simulink model "Group44PACEMAKER"  (R2022b)
settings: Solver=FixedStepAuto  StartTime=0.0  StopTime=2  FixedStep=1e-2  RelTol=1e-3  EnableMultiTasking=on
undefined symbols (not defined in the file): D0, D1, D10, D11, D12, D13, D2, D3, D4, D5, D6, D7, D8, D9, PTA0, PTA1, PTA2, PTB23, PTB9, PTC16, PTC17, PTC2, PTC3, PTC4, PTD0, PTD1, PTD2, PTD3
libraries: frdmk64flib x15, dsparch4 x1, dspstat3 x1
(part 1 of 2)
settings Model: ExtModeTrigDuration=5  Creator=Admin  LastModifiedBy=Admin
settings OptimizationCC: EnhancedBackFolding=on  PassReuseOutputArgsAs=Individual arguments  ZeroExternalMemoryAtStartup=off  ZeroInternalMemoryAtStartup=off  MaxStackSize=64  OptimizeBlockOrder=speed  DifferentSizesBufferReuse=on  OptimizationCustomize=off  EfficientTunableParamExpr=on
settings DebuggingCC: ParameterTunabilityLossMsg=error
settings HardwareCC: ProdBitPerPointer=32  ProdBitPerSizeT=32  ProdBitPerPtrDiffT=32  ProdLargestAtomicInteger=Long  ProdLargestAtomicFloat=Double  ProdWordSize=32  ProdHWDeviceType=ARM Compatible->ARM Cortex
settings SFSimCC: MATLABDynamicMemAlloc=off
settings RTWCC: Description=Embedded Coder  SystemTargetFile=ert.tlc  HardwareBoard=NXP FRDM-K64F  TLCOptions="-aInlineSetEventsForThisBaseRateFcn=TLC_FALSE -aSuppressMultiTaskScheduler=TLC_FALSE  -aRateBasedStepFcn=0"  TemplateMakefile=ert_default_tmf  Toolchain=GNU Tools for ARM Embedded Processors
settings CodeAppCC: ForceParamTrailComments=on  IgnoreCustomStorageClasses=off  OperatorAnnotations=on  SimulinkDataObjDesc=on  SFDataObjDesc=on  InsertBlockDesc=on
settings ERTTargetCC: ExtModeTransport=4  ExtModeMexFile=sendToCommService

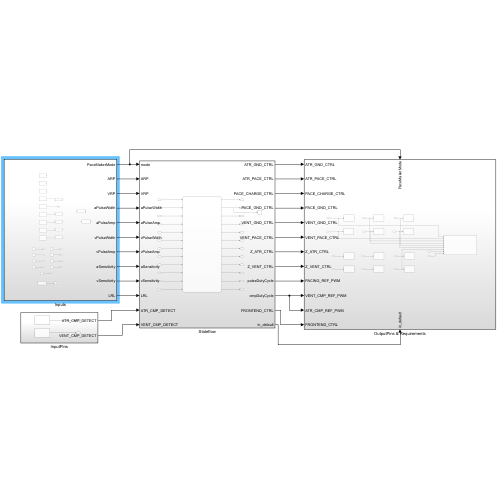
[thumbnail: Simulink's stored preview of the top-level diagram]
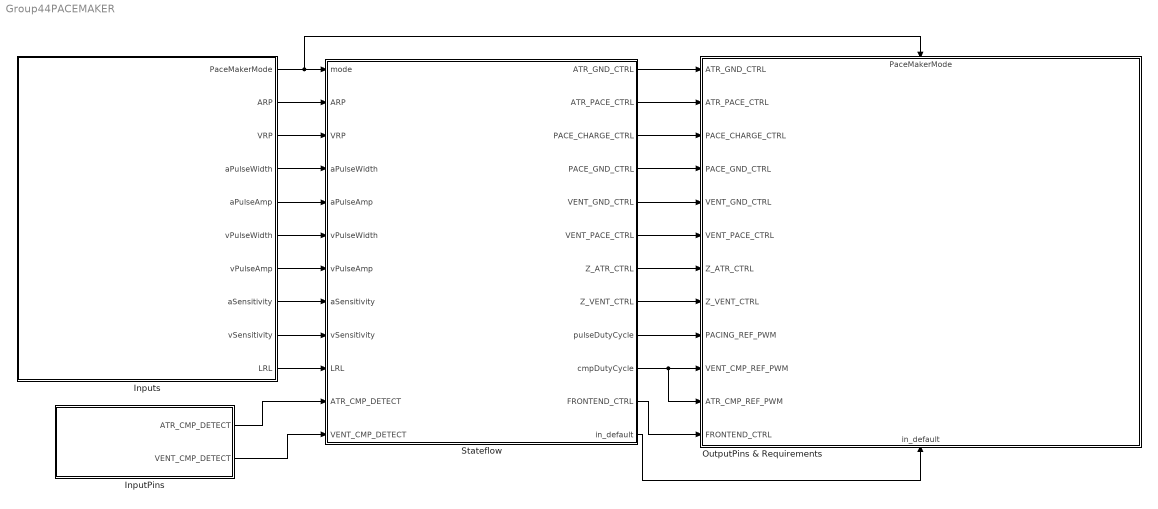
== system Group44PACEMAKER ==
  InputPins : Subsystem
  Inputs : Subsystem
  OutputPins & Requirements : Subsystem
      settings: PortSchema="{\"entries\":[{\"content\":{\"sides\":[{\"content\":{\"connectorIds\":[\"In1\",\"In2\",\"In3\",\"In4\",\"In5\",\"In6\",\"In7\",\"In8\",\"In9\",\"In10\",\"In11\",\"In12\"]},\"type\":\"ConnectorPlacement.EquallySpacedRectSide\",\"uuid\":\"f209b0ac-f79a-4701-a17d-e6e4657793a5\"},{\"content\":{\"connectorIds\":[],\"side\":\"RIGHT\"},\"type\":\"ConnectorPlacement.EquallySpacedRectSide\",\"uuid\":\"7d13a426-91e0-4712-bb01-5d8563f6962a\"},{\"content\":{\"connectorIds\":[\"In13\"],\"side\":\"TOP\"},\"type\":\"ConnectorPlacement.EquallySpacedRectSide\",\"uuid\":\"d5c2df9e-5684-45ec-bc45-fd2dab74cc87\"},{\"content\":{\"connectorIds\":[\"In14\"],\"side\":\"BOTTOM\"},\"type\":\"ConnectorPlacement.EquallySpacedRectSide\",\"uuid\":\"bae969d9-528a-49b4-ab28-7d9f0a0e5f3c\"}]},\"type\":\"ConnectorPlacement.EquallySpacedConnector\",\"uuid\":\"bb7a9bd2-ec42-4c9d-ad79-06266cd920c3\"}],\"packageUris\":[\"http://schema.mathworks.com/mf0/Connector/R2020b\"],\"version\":\"1.0\"}"
  Stateflow : Subsystem
  wires:
  Stateflow/12(in_default) -> OutputPins & Requirements/14(in_default)
  Stateflow/4(PACE_GND_CTRL) -> OutputPins & Requirements/4(PACE_GND_CTRL)
  Stateflow/10(cmpDutyCycle) -> OutputPins & Requirements/11(ATR_CMP_REF_PWM), OutputPins & Requirements/10(VENT_CMP_REF_PWM)
  Stateflow/5(VENT_GND_CTRL) -> OutputPins & Requirements/5(VENT_GND_CTRL)
  Stateflow/3(PACE_CHARGE_CTRL) -> OutputPins & Requirements/3(PACE_CHARGE_CTRL)
  InputPins/1(ATR_CMP_DETECT) -> Stateflow/11(ATR_CMP_DETECT)
  Stateflow/6(VENT_PACE_CTRL) -> OutputPins & Requirements/6(VENT_PACE_CTRL)
  Stateflow/2(ATR_PACE_CTRL) -> OutputPins & Requirements/2(ATR_PACE_CTRL)
  Stateflow/8(Z_VENT_CTRL) -> OutputPins & Requirements/8(Z_VENT_CTRL)
  Inputs/8(aSensitivity) -> Stateflow/8(aSensitivity)
  Inputs/7(vPulseAmp) -> Stateflow/7(vPulseAmp)
  Stateflow/7(Z_ATR_CTRL) -> OutputPins & Requirements/7(Z_ATR_CTRL)
  InputPins/2(VENT_CMP_DETECT) -> Stateflow/12(VENT_CMP_DETECT)
  Inputs/10(LRL) -> Stateflow/10(LRL)
  Stateflow/9(pulseDutyCycle) -> OutputPins & Requirements/9(PACING_REF_PWM)
  Inputs/4(aPulseWidth) -> Stateflow/4(aPulseWidth)
  Inputs/9(vSensitivity) -> Stateflow/9(vSensitivity)
  Inputs/2(ARP) -> Stateflow/2(ARP)
  Inputs/1(PaceMakerMode) -> OutputPins & Requirements/13(PaceMakerMode), Stateflow/1(mode)
  Stateflow/11(FRONTEND_CTRL) -> OutputPins & Requirements/12(FRONTEND_CTRL)
  Inputs/3(VRP) -> Stateflow/3(VRP)
  Inputs/6(vPulseWidth) -> Stateflow/6(vPulseWidth)
  Stateflow/1(ATR_GND_CTRL) -> OutputPins & Requirements/1(ATR_GND_CTRL)
  Inputs/5(aPulseAmp) -> Stateflow/5(aPulseAmp)

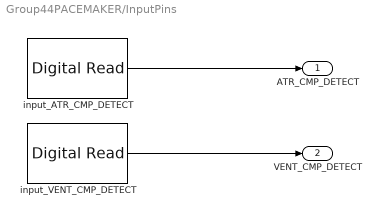
== system Group44PACEMAKER/InputPins ==
  input_ATR_CMP_DETECT : frdmk64flib/Digital Read  Whichpin=PTC16 (D0)  SampleTime=-1
  input_VENT_CMP_DETECT : frdmk64flib/Digital Read  Whichpin=PTC17 (D1)  SampleTime=-1
  ATR_CMP_DETECT : Outport  OutDataTypeStr=boolean
  VENT_CMP_DETECT : Outport  Port=2  OutDataTypeStr=boolean
  wires:
  input_ATR_CMP_DETECT/1 -> ATR_CMP_DETECT/1
  input_VENT_CMP_DETECT/1 -> VENT_CMP_DETECT/1

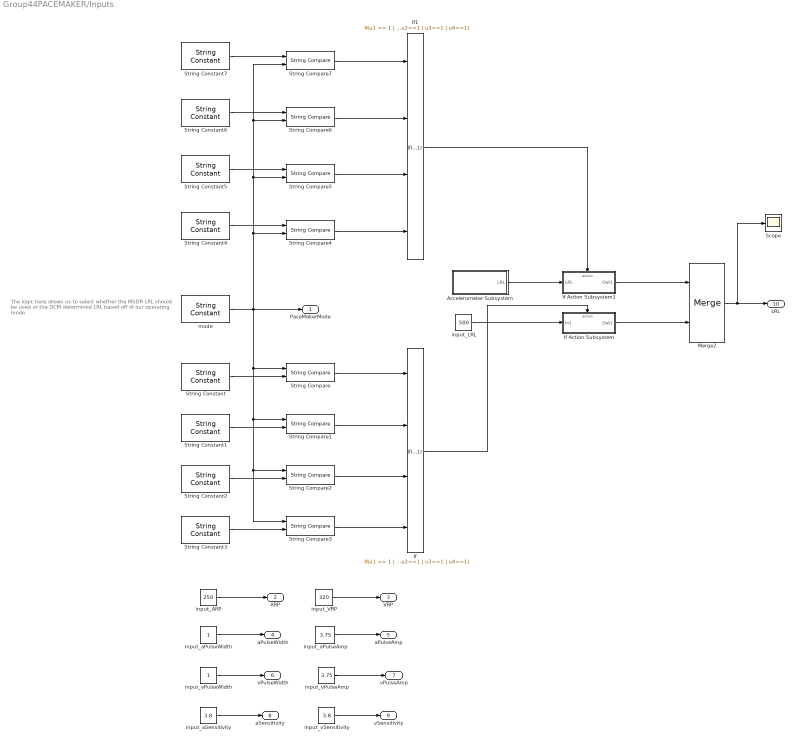
== system Group44PACEMAKER/Inputs ==
  note: The logic here allows us to select whether the MSDR LRL should be used or the DCM determined LRL based off of our operating mode
  Accelerometer Subsystem : Subsystem
  If : If  NumInputs=4  IfExpression=u1 == 1 | u2==1 | u3==1 | u4==1  ShowElse=off
  If Action Subsystem : Subsystem  TreatAsAtomicUnit=on
  If Action Subsystem1 : Subsystem  TreatAsAtomicUnit=on
  If1 : If  NumInputs=4  IfExpression=u1 == 1 | u2==1 | u3==1 | u4==1  ShowElse=off
  Merge2 : Merge
  Scope : Scope
  String Compare{,1..7} (8 alike) : StringCompare
  String Constant : StringConstant  String="\"AOO\""
  String Constant1 : StringConstant  String="\"AAI\""
  String Constant2 : StringConstant  String="\"VOO\""
  String Constant3 : StringConstant  String="\"VVI\""
  String Constant4 : StringConstant  String="\"AOOR\""
  String Constant5 : StringConstant  String="\"AAIR\""
  String Constant6 : StringConstant  String="\"VOOR\""
  String Constant7 : StringConstant  String="\"VVIR\""
  input_ARP : Constant  Value=250  OutDataTypeStr=double
  input_LRL : Constant  Value=500  OutDataTypeStr=double
  input_VRP : Constant  Value=320  OutDataTypeStr=double
  input_aPulseAmp : Constant  Value=3.75  OutDataTypeStr=double
  input_aPulseWidth : Constant  OutDataTypeStr=double
  input_aSensitivity : Constant  Value=3.8  OutDataTypeStr=double
  input_vPulseAmp : Constant  Value=3.75  OutDataTypeStr=double
  input_vPulseWidth : Constant  OutDataTypeStr=double
  input_vSensitivity : Constant  Value=3.8  OutDataTypeStr=double
  mode : StringConstant  String="\"AOOR\""
  PaceMakerMode : Outport  OutDataTypeStr=string
  ARP : Outport  Port=2  OutDataTypeStr=double  Unit=msec
  VRP : Outport  Port=3  OutDataTypeStr=double  Unit=msec
  aPulseWidth : Outport  Port=4  OutDataTypeStr=double  Unit=msec
  aPulseAmp : Outport  Port=5  OutDataTypeStr=double  Unit=V
  vPulseWidth : Outport  Port=6  OutDataTypeStr=double  Unit=msec
  vPulseAmp : Outport  Port=7  OutDataTypeStr=double  Unit=V
  aSensitivity : Outport  Port=8  OutDataTypeStr=double  Unit=V
  vSensitivity : Outport  Port=9  OutDataTypeStr=double  Unit=V
  LRL : Outport  Port=10  OutDataTypeStr=double  Unit=msec
  wires:
  mode/1 -> String Compare7/2, String Compare6/2, String Compare5/2, String Compare4/2, String Compare1/1, String Compare2/1, String Compare3/1, String Compare/1, PaceMakerMode/1
  input_aPulseAmp/1 -> aPulseAmp/1
  input_ARP/1 -> ARP/1
  input_VRP/1 -> VRP/1
  input_aPulseWidth/1 -> aPulseWidth/1
  input_vPulseWidth/1 -> vPulseWidth/1
  input_vPulseAmp/1 -> vPulseAmp/1
  input_vSensitivity/1 -> vSensitivity/1
  input_aSensitivity/1 -> aSensitivity/1
  String Constant/1 -> String Compare/2
  String Constant1/1 -> String Compare1/2
  String Constant2/1 -> String Compare2/2
  String Constant3/1 -> String Compare3/2
  String Constant4/1 -> String Compare4/1
  String Constant5/1 -> String Compare5/1
  String Constant6/1 -> String Compare6/1
  String Constant7/1 -> String Compare7/1
  If/1 -> If Action Subsystem/Action
  input_LRL/1 -> If Action Subsystem/1(In1)
  Merge2/1 -> Scope/1, LRL/1
  If Action Subsystem/1(Out1) -> Merge2/2
  If Action Subsystem1/1(Out1) -> Merge2/1
  String Compare3/1 -> If/4
  String Compare2/1 -> If/3
  String Compare1/1 -> If/2
  String Compare/1 -> If/1
  Accelerometer Subsystem/1(LRL) -> If Action Subsystem1/1(LRL)
  String Compare7/1 -> If1/1
  String Compare6/1 -> If1/2
  String Compare5/1 -> If1/3
  String Compare4/1 -> If1/4
  If1/1 -> If Action Subsystem1/Action

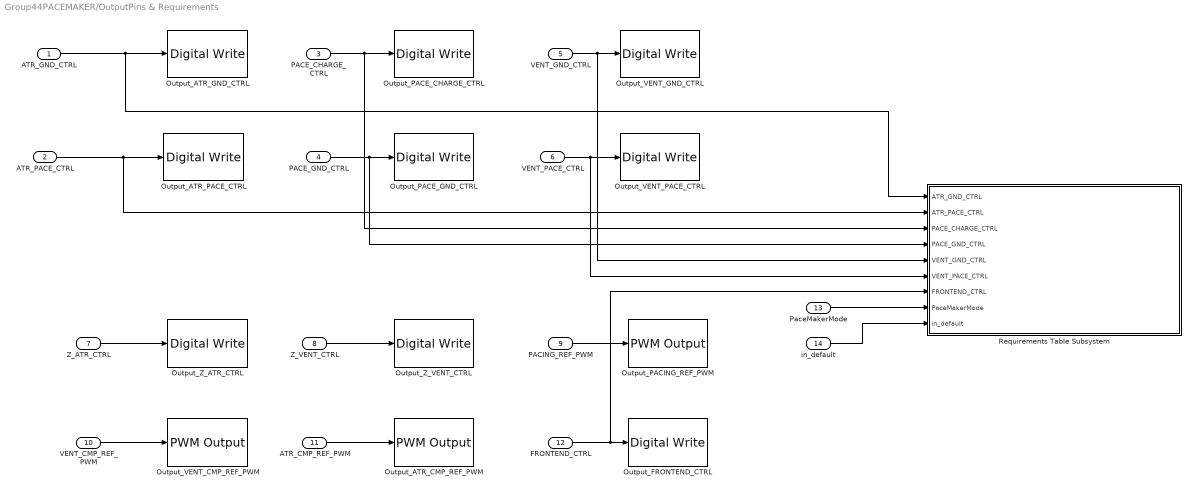
== system Group44PACEMAKER/OutputPins & Requirements ==
  ATR_GND_CTRL : Inport  OutDataTypeStr=boolean
  ATR_PACE_CTRL : Inport  Port=2  OutDataTypeStr=boolean
  PACE_CHARGE_CTRL : Inport  Port=3  OutDataTypeStr=boolean
  PACE_GND_CTRL : Inport  Port=4  OutDataTypeStr=boolean
  VENT_GND_CTRL : Inport  Port=5  OutDataTypeStr=boolean
  VENT_PACE_CTRL : Inport  Port=6  OutDataTypeStr=boolean
  Z_ATR_CTRL : Inport  Port=7  OutDataTypeStr=boolean
  Z_VENT_CTRL : Inport  Port=8  OutDataTypeStr=boolean
  PACING_REF_PWM : Inport  Port=9  OutDataTypeStr=double
  VENT_CMP_REF_PWM : Inport  Port=10  OutDataTypeStr=double
  ATR_CMP_REF_PWM : Inport  Port=11  OutDataTypeStr=double
  FRONTEND_CTRL : Inport  Port=12  OutDataTypeStr=boolean
  PaceMakerMode : Inport  Port=13  OutDataTypeStr=string
  in_default : Inport  Port=14  OutDataTypeStr=boolean
  Output_ATR_CMP_REF_PWM : frdmk64flib/PWM Output  Whichpin=PTC2 (D6)  InitialFrequency=2000  InitialDutyCycle=0
  Output_ATR_GND_CTRL : frdmk64flib/Digital Write  Whichpin=PTD2 (D11)
  Output_ATR_PACE_CTRL : frdmk64flib/Digital Write  Whichpin=PTA0 (D8)
  Output_FRONTEND_CTRL : frdmk64flib/Digital Write  Whichpin=PTD1 (D13)
  Output_PACE_CHARGE_CTRL : frdmk64flib/Digital Write  Whichpin=PTB9 (D2)
  Output_PACE_GND_CTRL : frdmk64flib/Digital Write  Whichpin=PTD0 (D10)
  Output_PACING_REF_PWM : frdmk64flib/PWM Output  Whichpin=PTA2 (D5)  InitialFrequency=2000  InitialDutyCycle=0
  Output_VENT_CMP_REF_PWM : frdmk64flib/PWM Output  Whichpin=PTA1 (D3)  InitialFrequency=2000  InitialDutyCycle=0
  Output_VENT_GND_CTRL : frdmk64flib/Digital Write  Whichpin=PTD3 (D12)
  Output_VENT_PACE_CTRL : frdmk64flib/Digital Write  Whichpin=PTC4 (D9)
  Output_Z_ATR_CTRL : frdmk64flib/Digital Write  Whichpin=PTB23 (D4)
  Output_Z_VENT_CTRL : frdmk64flib/Digital Write  Whichpin=PTC3 (D7)
  Requirements Table Subsystem : Subsystem
  wires:
  ATR_GND_CTRL/1 -> Requirements Table Subsystem/1(ATR_GND_CTRL), Output_ATR_GND_CTRL/1
  PACE_CHARGE_CTRL/1 -> Requirements Table Subsystem/3(PACE_CHARGE_CTRL), Output_PACE_CHARGE_CTRL/1
  VENT_GND_CTRL/1 -> Requirements Table Subsystem/5(VENT_GND_CTRL), Output_VENT_GND_CTRL/1
  VENT_PACE_CTRL/1 -> Requirements Table Subsystem/6(VENT_PACE_CTRL), Output_VENT_PACE_CTRL/1
  PACE_GND_CTRL/1 -> Requirements Table Subsystem/4(PACE_GND_CTRL), Output_PACE_GND_CTRL/1
  ATR_PACE_CTRL/1 -> Requirements Table Subsystem/2(ATR_PACE_CTRL), Output_ATR_PACE_CTRL/1
  Z_ATR_CTRL/1 -> Output_Z_ATR_CTRL/1
  Z_VENT_CTRL/1 -> Output_Z_VENT_CTRL/1
  PACING_REF_PWM/1 -> Output_PACING_REF_PWM/1
  ATR_CMP_REF_PWM/1 -> Output_ATR_CMP_REF_PWM/1
  VENT_CMP_REF_PWM/1 -> Output_VENT_CMP_REF_PWM/1
  FRONTEND_CTRL/1 -> Output_FRONTEND_CTRL/1, Requirements Table Subsystem/7(FRONTEND_CTRL)
  PaceMakerMode/1 -> Requirements Table Subsystem/8(PaceMakerMode)
  in_default/1 -> Requirements Table Subsystem/9(in_default)

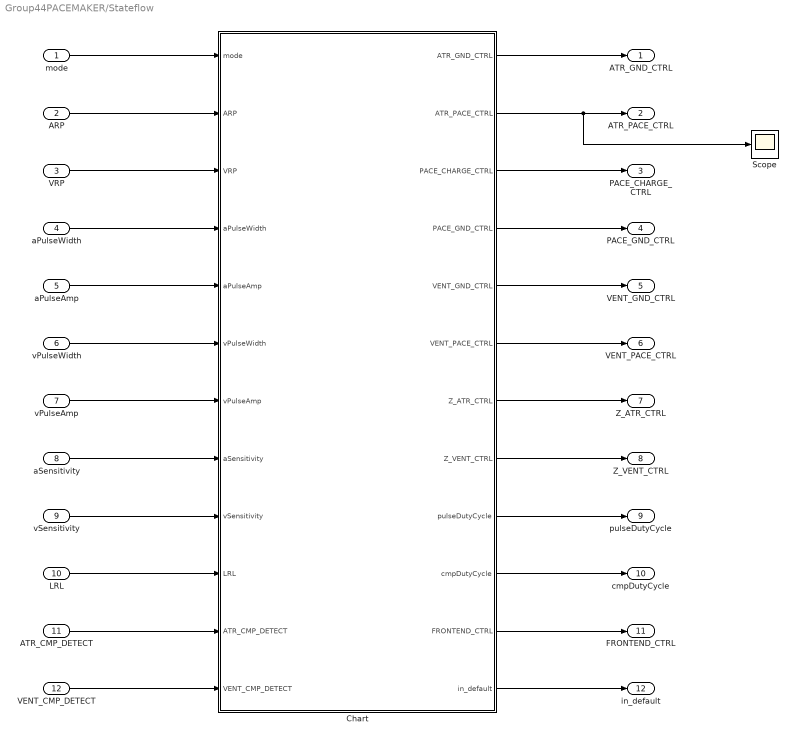
== system Group44PACEMAKER/Stateflow ==
  mode : Inport  OutDataTypeStr=string
  ARP : Inport  Port=2  OutDataTypeStr=double  Unit=msec
  VRP : Inport  Port=3  OutDataTypeStr=double  Unit=msec
  aPulseWidth : Inport  Port=4  OutDataTypeStr=double  Unit=msec
  aPulseAmp : Inport  Port=5  OutDataTypeStr=double  Unit=V
  vPulseWidth : Inport  Port=6  OutDataTypeStr=double  Unit=msec
  vPulseAmp : Inport  Port=7  OutDataTypeStr=double  Unit=V
  aSensitivity : Inport  Port=8  OutDataTypeStr=double  Unit=V
  vSensitivity : Inport  Port=9  OutDataTypeStr=double  Unit=V
  LRL : Inport  Port=10  OutDataTypeStr=double  Unit=msec
  ATR_CMP_DETECT : Inport  Port=11  OutDataTypeStr=boolean
  VENT_CMP_DETECT : Inport  Port=12  OutDataTypeStr=boolean
  Chart : Stateflow chart  TreatAsAtomicUnit=on
      settings: PortSchema="{\"entries\":[{\"content\":{\"sides\":[{\"content\":{\"connectorIds\":[\"In1\",\"In2\",\"In3\",\"In4\",\"In5\",\"In6\",\"In7\",\"In8\",\"In9\",\"In10\",\"In11\",\"In12\"]},\"type\":\"ConnectorPlacement.EquallySpacedRectSide\",\"uuid\":\"859ad6b1-f88a-4c7a-b788-dab0771a046c\"},{\"content\":{\"connectorIds\":[\"Out1\",\"Out2\",\"Out4\",\"Out5\",\"Out6\",\"Out7\",\"Out8\",\"Out9\",\"Out12\",\"Out10\",\"Out3\",\"Out11\"],\"side\":\"RIGHT\"},\"type\":\"ConnectorPlacement.EquallySpacedRectSide\",\"uuid\":\"6cbb226c-0635-41e8-91ac-a9d01d96dd8d\"},{\"content\":{\"connectorIds\":[],\"side\":\"TOP\"},\"type\":\"ConnectorPlacement.EquallySpacedRectSide\",\"uuid\":\"47ebdae6-f6ae-4f62-b33d-fff46319b1f0\"}]},\"type\":\"ConnectorPlacement.EquallySpacedConnector\",\"uuid\":\"c5e573a1-920d-4865-9b5e-320d436c45e0\"}],\"packageUris\":[\"http://schema.mathworks.com/mf0/Connector/R2020b\"],\"version\":\"1.0\"}"
  Scope : Scope
  ATR_GND_CTRL : Outport  OutDataTypeStr=boolean
  ATR_PACE_CTRL : Outport  Port=2  OutDataTypeStr=boolean
  PACE_CHARGE_CTRL : Outport  Port=3  OutDataTypeStr=boolean
  PACE_GND_CTRL : Outport  Port=4  OutDataTypeStr=boolean
  VENT_GND_CTRL : Outport  Port=5  OutDataTypeStr=boolean
  VENT_PACE_CTRL : Outport  Port=6  OutDataTypeStr=boolean
  Z_ATR_CTRL : Outport  Port=7  OutDataTypeStr=boolean
  Z_VENT_CTRL : Outport  Port=8  OutDataTypeStr=boolean
  pulseDutyCycle : Outport  Port=9  OutDataTypeStr=double
  cmpDutyCycle : Outport  Port=10  OutDataTypeStr=double
  FRONTEND_CTRL : Outport  Port=11  OutDataTypeStr=boolean
  in_default : Outport  Port=12  OutDataTypeStr=boolean
  wires:
  mode/1 -> Chart/1(mode)
  ARP/1 -> Chart/2(ARP)
  VRP/1 -> Chart/3(VRP)
  aPulseWidth/1 -> Chart/4(aPulseWidth)
  aPulseAmp/1 -> Chart/5(aPulseAmp)
  vPulseWidth/1 -> Chart/6(vPulseWidth)
  vPulseAmp/1 -> Chart/7(vPulseAmp)
  aSensitivity/1 -> Chart/8(aSensitivity)
  vSensitivity/1 -> Chart/9(vSensitivity)
  LRL/1 -> Chart/10(LRL)
  ATR_CMP_DETECT/1 -> Chart/11(ATR_CMP_DETECT)
  VENT_CMP_DETECT/1 -> Chart/12(VENT_CMP_DETECT)
  Chart/1(ATR_GND_CTRL) -> ATR_GND_CTRL/1
  Chart/2(ATR_PACE_CTRL) -> Scope/1, ATR_PACE_CTRL/1
  Chart/4(PACE_CHARGE_CTRL) -> PACE_CHARGE_CTRL/1
  Chart/5(PACE_GND_CTRL) -> PACE_GND_CTRL/1
  Chart/6(VENT_GND_CTRL) -> VENT_GND_CTRL/1
  Chart/7(VENT_PACE_CTRL) -> VENT_PACE_CTRL/1
  Chart/8(Z_ATR_CTRL) -> Z_ATR_CTRL/1
  Chart/9(Z_VENT_CTRL) -> Z_VENT_CTRL/1
  Chart/10(cmpDutyCycle) -> cmpDutyCycle/1
  Chart/3(FRONTEND_CTRL) -> FRONTEND_CTRL/1
  Chart/11(in_default) -> in_default/1
  Chart/12(pulseDutyCycle) -> pulseDutyCycle/1

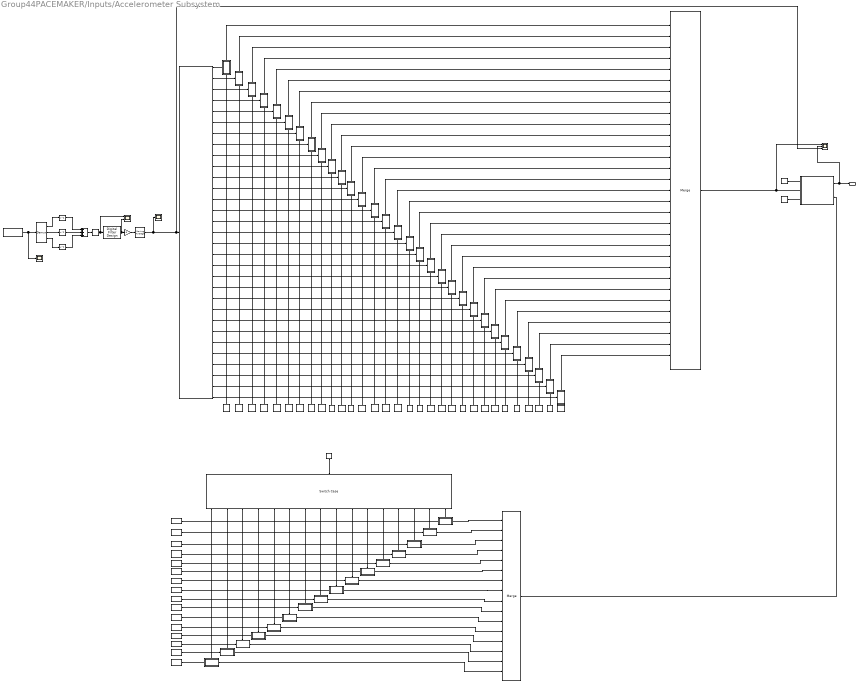
== system Group44PACEMAKER/Inputs/Accelerometer Subsystem ==
  note: The chart allows us to come up with a steady rate of change for the heart LRL such that the heart rate changes smoothly over the reaction time/recovery time
  note: This if else block allows us to select the appropriate LRL based on activity level
  note: The squared terms, adder, and square root term allow us to get the magnitude of the acceleration vector
  note: Moving average smooths out activity level and allows us to average out the activity for the past x seconds dependent of model fixed step time and the window used
  note: The gain function amplifies the signal so changes in activity can easily be observed using the scope
  note: The low pass filter gets rid of any intense spikes or dips that are not characterist of the activity
  note: The response factor can range from 1 to 16. 1 being the lowest response factor and 16 being the highest.
      | The response factor is used to determine a percentage of the of the reaction time that will be used to adjust the LRL. (Eg, a response factor of 1 will use 100% of the reaction time however a response factor of 16 will only use 70% of the reaction time)
  100 bpm : Constant  Value=600
  105 bpm : Constant  Value=571.43
  110 bpm : Constant  Value=545.45
  115 bpm : Constant  Value=521.74
  120 bpm : Constant  Value=500
  125 bpm : Constant  Value=480
  130 bpm : Constant  Value=461.54
  135 bpm : Constant  Value=444.44
  140 bpm : Constant  Value=428.57
  145 bpm : Constant  Value=413.79
  150 bpm : Constant  Value=400
  155 bpm : Constant  Value=387.10
  160 bpm : Constant  Value=375
  165 bpm : Constant  Value=363.63
  170 bpm1 : Constant  Value=352.94
  175 bpm : Constant  Value=342.86
  180 bpm : Constant  Value=333.33
  185 bpm : Constant  Value=324.32
  190 bpm : Constant  Value=315.79
  195 bpm : Constant  Value=307.69
  200 bpm : Constant  Value=300
  205 bpm : Constant  Value=292.68
  55 bpm : Constant  Value=1090.91
  60 bpm : Constant  Value=1000
  65 bpm : Constant  Value=923.08
  70 bpm : Constant  Value=857.14
  75 bpm : Constant  Value=800
  80 bpm : Constant  Value=750
  85 bpm : Constant  Value=705.88
  90 bpm : Constant  Value=666.67
  95 bpm : Constant  Value=631.58
  >7.9 : Subsystem  TreatAsAtomicUnit=on
  >8 : Subsystem  TreatAsAtomicUnit=on
  Accelerometer : Subsystem
  Add : Sum  Inputs=+++
  Change LRL Smoothly : Stateflow chart  TreatAsAtomicUnit=on
      settings: PortSchema="{\"entries\":[{\"content\":{\"sides\":[{\"content\":{\"connectorIds\":[\"In3\",\"In2\",\"In4\"]},\"type\":\"ConnectorPlacement.EquallySpacedRectSide\",\"uuid\":\"85af1beb-61ae-4766-b408-8225321ec4a4\"},{\"content\":{\"connectorIds\":[\"Out1\",\"In1\"],\"side\":\"RIGHT\"},\"type\":\"ConnectorPlacement.EquallySpacedRectSide\",\"uuid\":\"bdf3d147-5894-49ca-bdec-54ebdf64bfa8\"},{\"content\":{\"connectorIds\":[],\"side\":\"TOP\"},\"type\":\"ConnectorPlacement.EquallySpacedRectSide\",\"uuid\":\"42bc5e47-54de-4fed-b1f0-fe2ea6e0cd28\"},{\"content\":{\"connectorIds\":[],\"side\":\"BOTTOM\"},\"type\":\"ConnectorPlacement.EquallySpacedRectSide\",\"uuid\":\"092d377f-872f-4731-90ca-5dcd29f87b08\"}]},\"type\":\"ConnectorPlacement.EquallySpacedConnector\",\"uuid\":\"a2c4c5d6-6aa5-4141-8747-f931ac594277\"}],\"packageUris\":[\"http://schema.mathworks.com/mf0/Connector/R2020b\"],\"version\":\"1.0\"}"
  Demux : Demux  Outputs=3
      settings: DisplayOption=none
  Gain : Gain  Gain=5
  If : If  IfExpression=u1 > 8  ElseIfExpressions=u1>7.9, u1>7.8, u1>7.7, u1>7.6, u1>7.5, u1>7.4, u1>7.3, u1>7.2, u1>7.1, u1 > 7, u1>6.9, u1>6.8, u1>6.7, u1>6.6, u1>6.5, u1>6.4, u1>6.3, u1>6.2, u1>6.1, u1 >6, u1>5.9, u1>5.8, u1>5.7, u1>5.6, u1>5.5, u1>5.4, u1>5.3, u1>5.2, u1>5.1
  If Action Subsystem : Subsystem  TreatAsAtomicUnit=on
  If Action Subsystem1 : Subsystem  TreatAsAtomicUnit=on
  If Action Subsystem10 : Subsystem  TreatAsAtomicUnit=on
  If Action Subsystem11 : Subsystem  TreatAsAtomicUnit=on
  If Action Subsystem12 : Subsystem  TreatAsAtomicUnit=on
  If Action Subsystem13 : Subsystem  TreatAsAtomicUnit=on
  If Action Subsystem14 : Subsystem  TreatAsAtomicUnit=on
  If Action Subsystem15 : Subsystem  TreatAsAtomicUnit=on
  If Action Subsystem16 : Subsystem  TreatAsAtomicUnit=on
  If Action Subsystem17 : Subsystem  TreatAsAtomicUnit=on
  If Action Subsystem18 : Subsystem  TreatAsAtomicUnit=on
  If Action Subsystem19 : Subsystem  TreatAsAtomicUnit=on
  If Action Subsystem2 : Subsystem  TreatAsAtomicUnit=on
  If Action Subsystem20 : Subsystem  TreatAsAtomicUnit=on
  If Action Subsystem21 : Subsystem  TreatAsAtomicUnit=on
  If Action Subsystem22 : Subsystem  TreatAsAtomicUnit=on
  If Action Subsystem23 : Subsystem  TreatAsAtomicUnit=on
  If Action Subsystem24 : Subsystem  TreatAsAtomicUnit=on
  If Action Subsystem25 : Subsystem  TreatAsAtomicUnit=on
  If Action Subsystem26 : Subsystem  TreatAsAtomicUnit=on
  If Action Subsystem3 : Subsystem  TreatAsAtomicUnit=on
  If Action Subsystem4 : Subsystem  TreatAsAtomicUnit=on
  If Action Subsystem5 : Subsystem  TreatAsAtomicUnit=on
  If Action Subsystem6 : Subsystem  TreatAsAtomicUnit=on
  If Action Subsystem7 : Subsystem  TreatAsAtomicUnit=on
  If Action Subsystem8 : Subsystem  TreatAsAtomicUnit=on
  If Action Subsystem9 : Subsystem  TreatAsAtomicUnit=on
  LowPassFilter : dsparch4/Digital Filter Design  mwdsp_browser_bugfix_var=off
  Merge : Merge  Inputs=31
  Merge1 : Merge  Inputs=16
  Moderate activity LRL if subsystem : Subsystem  TreatAsAtomicUnit=on
  Moving Average1 : dspstat3/Moving Average  Method=Sliding window  ForgettingFactorPort=off  SpecifyWindowLength=on  WindowLength=500  OverlapLength=499  AllowArbitraryInputLength=off  ForgettingFactor=0.9  SimulateUsing=Code generation
  RF == 1 : Subsystem  TreatAsAtomicUnit=on
  RF == 10 : Subsystem  TreatAsAtomicUnit=on
  RF == 11 : Subsystem  TreatAsAtomicUnit=on
  RF == 12 : Subsystem  TreatAsAtomicUnit=on
  RF == 13 : Subsystem  TreatAsAtomicUnit=on
  RF == 14 : Subsystem  TreatAsAtomicUnit=on
  RF == 15 : Subsystem  TreatAsAtomicUnit=on
  RF == 16 : Subsystem  TreatAsAtomicUnit=on
  RF == 2 : Subsystem  TreatAsAtomicUnit=on
  RF == 3 : Subsystem  TreatAsAtomicUnit=on
  RF == 4 : Subsystem  TreatAsAtomicUnit=on
  RF == 5 : Subsystem  TreatAsAtomicUnit=on
  RF == 6 : Subsystem  TreatAsAtomicUnit=on
  RF == 7 : Subsystem  TreatAsAtomicUnit=on
  RF == 8 : Subsystem  TreatAsAtomicUnit=on
  RF == 9 : Subsystem  TreatAsAtomicUnit=on
  RF_1 : Constant  Value=100
  RF_10 : Constant  Value=82
  RF_11 : Constant  Value=80
  RF_12 : Constant  Value=78
  RF_13 : Constant  Value=76
  RF_14 : Constant  Value=74
  RF_15 : Constant  Value=72
  RF_16 : Constant  Value=70
  RF_2 : Constant  Value=98  OutDataTypeStr=double
  RF_3 : Constant  Value=96
  RF_4 : Constant  Value=94
  RF_5 : Constant  Value=92
  RF_6 : Constant  Value=90
  RF_7 : Constant  Value=88
  RF_8 : Constant  Value=86
  RF_9 : Constant  Value=84
  Response Factor Switch Case : SwitchCase  CaseConditions={1,2,3,4,5,6,7,8,9,10,11,12,13,14,15,16}  ShowDefaultCase=off
  Response_factor : Constant
  Scope : Scope  NumInputPorts=3
  Scope1 : Scope
  Scope2 : Scope  NumInputPorts=2
  Scope3 : Scope
  Square : Math  Operator=square
  Square Root : Sqrt
  Square1 : Math  Operator=square
  Square2 : Math  Operator=square
  Vigorous activity LRL if subsystem : Subsystem  TreatAsAtomicUnit=on
  reaction_time(sec) : Constant  Value=5
  recovery_time(min) : Constant  Value=.1
  LRL : Outport
  wires:
  Add/1 -> Square Root/1
  Gain/1 -> Moving Average1/1
  Square1/1 -> Add/2
  LowPassFilter/1 -> Scope2/2, Gain/1
  Square/1 -> Add/1
  Demux/2 -> Square1/1
  Accelerometer/1(Acceleration) -> Scope1/1, Demux/1
  Demux/3 -> Square2/1
  Demux/1 -> Square/1
  Square2/1 -> Add/3
  Square Root/1 -> Scope2/1, LowPassFilter/1
  Moving Average1/1 -> Scope3/1, Scope/3, If/1
  Merge/1 -> Scope/1, Change LRL Smoothly/2(inputLRL)
  Change LRL Smoothly/1(outputLRL) -> LRL/1, Scope/2
  reaction_time(sec)/1 -> Change LRL Smoothly/3(reaction_time)
  recovery_time(min)/1 -> Change LRL Smoothly/4(recovery_time)
  Response_factor/1 -> Response Factor Switch Case/1
  Response Factor Switch Case/2 -> RF == 2/Action
  Response Factor Switch Case/1 -> RF == 1/Action
  Response Factor Switch Case/3 -> RF == 3/Action
  Response Factor Switch Case/4 -> RF == 4/Action
  Response Factor Switch Case/5 -> RF == 5/Action
  Response Factor Switch Case/6 -> RF == 6/Action
  Response Factor Switch Case/7 -> RF == 7/Action
  Response Factor Switch Case/8 -> RF == 8/Action
  Response Factor Switch Case/9 -> RF == 9/Action
  Response Factor Switch Case/10 -> RF == 10/Action
  Response Factor Switch Case/11 -> RF == 11/Action
  Response Factor Switch Case/12 -> RF == 12/Action
  Response Factor Switch Case/13 -> RF == 13/Action
  Response Factor Switch Case/15 -> RF == 15/Action
  Response Factor Switch Case/14 -> RF == 14/Action
  Response Factor Switch Case/16 -> RF == 16/Action
  RF_1/1 -> RF == 1/1(In1)
  RF_3/1 -> RF == 3/1(In1)
  RF_2/1 -> RF == 2/1(In1)
  RF_4/1 -> RF == 4/1(In1)
  RF_5/1 -> RF == 5/1(In1)
  RF_6/1 -> RF == 6/1(In1)
  RF_7/1 -> RF == 7/1(In1)
  RF_8/1 -> RF == 8/1(In1)
  RF_9/1 -> RF == 9/1(In1)
  RF_10/1 -> RF == 10/1(In1)
  RF_11/1 -> RF == 11/1(In1)
  RF_12/1 -> RF == 12/1(In1)
  RF_13/1 -> RF == 13/1(In1)
  RF_14/1 -> RF == 14/1(In1)
  RF_15/1 -> RF == 15/1(In1)
  RF_16/1 -> RF == 16/1(In1)
  RF == 16/1(Out1) -> Merge1/1
  RF == 15/1(Out1) -> Merge1/2
  RF == 14/1(Out1) -> Merge1/3
  RF == 13/1(Out1) -> Merge1/4
  RF == 12/1(Out1) -> Merge1/5
  RF == 11/1(Out1) -> Merge1/6
  RF == 10/1(Out1) -> Merge1/7
  RF == 1/1(Out1) -> Merge1/16
  RF == 2/1(Out1) -> Merge1/15
  RF == 3/1(Out1) -> Merge1/14
  RF == 4/1(Out1) -> Merge1/13
  RF == 5/1(Out1) -> Merge1/12
  RF == 6/1(Out1) -> Merge1/11
  RF == 7/1(Out1) -> Merge1/10
  RF == 8/1(Out1) -> Merge1/9
  RF == 9/1(Out1) -> Merge1/8
  Merge1/1 -> Change LRL Smoothly/1(Response_factor)
  If/1 -> >8/Action
  If/2 -> >7.9/Action
  If/3 -> Moderate activity LRL if subsystem/Action
  If/4 -> Vigorous activity LRL if subsystem/Action
  If/5 -> If Action Subsystem/Action
  If/6 -> If Action Subsystem1/Action
  If/7 -> If Action Subsystem2/Action
  If/8 -> If Action Subsystem3/Action
  If/9 -> If Action Subsystem4/Action
  If/10 -> If Action Subsystem5/Action
  If/11 -> If Action Subsystem6/Action
  If/12 -> If Action Subsystem7/Action
  If/13 -> If Action Subsystem8/Action
  If/14 -> If Action Subsystem9/Action
  If/15 -> If Action Subsystem10/Action
  If/16 -> If Action Subsystem11/Action
  If/17 -> If Action Subsystem12/Action
  If/18 -> If Action Subsystem13/Action
  If/19 -> If Action Subsystem14/Action
  If/20 -> If Action Subsystem15/Action
  If/21 -> If Action Subsystem16/Action
  If/22 -> If Action Subsystem17/Action
  If/23 -> If Action Subsystem18/Action
  If/24 -> If Action Subsystem19/Action
  If/25 -> If Action Subsystem20/Action
  If/26 -> If Action Subsystem21/Action
  If/27 -> If Action Subsystem22/Action
  If/28 -> If Action Subsystem23/Action
  If/29 -> If Action Subsystem24/Action
  If/30 -> If Action Subsystem25/Action
  If/31 -> If Action Subsystem26/Action
  205 bpm/1 -> >8/1(In1)
  200 bpm/1 -> >7.9/1(In1)
  195 bpm/1 -> Moderate activity LRL if subsystem/1(In1)
  190 bpm/1 -> Vigorous activity LRL if subsystem/1(In1)
  185 bpm/1 -> If Action Subsystem/1(In1)
  180 bpm/1 -> If Action Subsystem1/1(In1)
  175 bpm/1 -> If Action Subsystem2/1(In1)
  170 bpm1/1 -> If Action Subsystem3/1(In1)
  165 bpm/1 -> If Action Subsystem4/1(In1)
  160 bpm/1 -> If Action Subsystem5/1(In1)
  155 bpm/1 -> If Action Subsystem6/1(In1)
  150 bpm/1 -> If Action Subsystem7/1(In1)
  145 bpm/1 -> If Action Subsystem8/1(In1)
  140 bpm/1 -> If Action Subsystem9/1(In1)
  135 bpm/1 -> If Action Subsystem10/1(In1)
  130 bpm/1 -> If Action Subsystem11/1(In1)
  125 bpm/1 -> If Action Subsystem12/1(In1)
  120 bpm/1 -> If Action Subsystem13/1(In1)
  115 bpm/1 -> If Action Subsystem14/1(In1)
  110 bpm/1 -> If Action Subsystem15/1(In1)
  105 bpm/1 -> If Action Subsystem16/1(In1)
  100 bpm/1 -> If Action Subsystem17/1(In1)
  95 bpm/1 -> If Action Subsystem18/1(In1)
  90 bpm/1 -> If Action Subsystem19/1(In1)
  85 bpm/1 -> If Action Subsystem20/1(In1)
  80 bpm/1 -> If Action Subsystem21/1(In1)
  75 bpm/1 -> If Action Subsystem22/1(In1)
  70 bpm/1 -> If Action Subsystem23/1(In1)
  65 bpm/1 -> If Action Subsystem24/1(In1)
  60 bpm/1 -> If Action Subsystem25/1(In1)
  55 bpm/1 -> If Action Subsystem26/1(In1)
  >8/1(Out1) -> Merge/1
  >7.9/1(Out1) -> Merge/2
  Moderate activity LRL if subsystem/1(Out1) -> Merge/3
  Vigorous activity LRL if subsystem/1(Out1) -> Merge/4
  If Action Subsystem/1(Out1) -> Merge/5
  If Action Subsystem1/1(Out1) -> Merge/6
  If Action Subsystem2/1(Out1) -> Merge/7
  If Action Subsystem3/1(Out1) -> Merge/8
  If Action Subsystem4/1(Out1) -> Merge/9
  If Action Subsystem5/1(Out1) -> Merge/10
  If Action Subsystem6/1(Out1) -> Merge/11
  If Action Subsystem7/1(Out1) -> Merge/12
  If Action Subsystem8/1(Out1) -> Merge/13
  If Action Subsystem9/1(Out1) -> Merge/14
  If Action Subsystem10/1(Out1) -> Merge/15
  If Action Subsystem11/1(Out1) -> Merge/16
  If Action Subsystem12/1(Out1) -> Merge/17
  If Action Subsystem13/1(Out1) -> Merge/18
  If Action Subsystem14/1(Out1) -> Merge/19
  If Action Subsystem15/1(Out1) -> Merge/20
  If Action Subsystem16/1(Out1) -> Merge/21
  If Action Subsystem17/1(Out1) -> Merge/22
  If Action Subsystem18/1(Out1) -> Merge/23
  If Action Subsystem19/1(Out1) -> Merge/24
  If Action Subsystem20/1(Out1) -> Merge/25
  If Action Subsystem21/1(Out1) -> Merge/26
  If Action Subsystem22/1(Out1) -> Merge/27
  If Action Subsystem23/1(Out1) -> Merge/28
  If Action Subsystem24/1(Out1) -> Merge/29
  If Action Subsystem25/1(Out1) -> Merge/30
  If Action Subsystem26/1(Out1) -> Merge/31

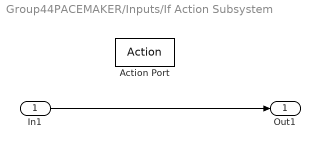
== system Group44PACEMAKER/Inputs/If Action Subsystem ==
  In1 : Inport
  Action Port : ActionPort  ActionPortLabel=if(u1 == 1 | u2==1 | u3==1 | u4==1)
  Out1 : Outport
  wires:
  In1/1 -> Out1/1

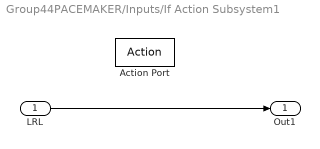
== system Group44PACEMAKER/Inputs/If Action Subsystem1 ==
  LRL : Inport
  Action Port : ActionPort  ActionPortLabel=if(u1 == 1 | u2==1 | u3==1 | u4==1)
  Out1 : Outport
  wires:
  LRL/1 -> Out1/1

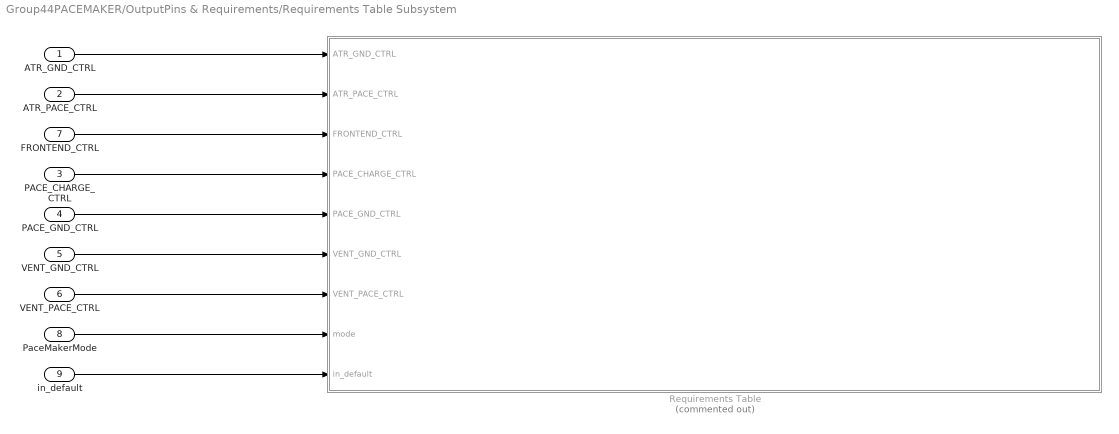
== system Group44PACEMAKER/OutputPins & Requirements/Requirements Table Subsystem ==
  ATR_GND_CTRL : Inport  OutDataTypeStr=boolean
  ATR_PACE_CTRL : Inport  Port=2  OutDataTypeStr=boolean
  PACE_CHARGE_CTRL : Inport  Port=3  OutDataTypeStr=boolean
  PACE_GND_CTRL : Inport  Port=4  OutDataTypeStr=boolean
  VENT_GND_CTRL : Inport  Port=5  OutDataTypeStr=boolean
  VENT_PACE_CTRL : Inport  Port=6  OutDataTypeStr=boolean
  FRONTEND_CTRL : Inport  Port=7  OutDataTypeStr=boolean
  PaceMakerMode : Inport  Port=8  OutDataTypeStr=string
  in_default : Inport  Port=9  OutDataTypeStr=boolean
  Requirements Table : Requirements Table  Commented=on  TreatAsAtomicUnit=on
  wires:
  ATR_GND_CTRL/1 -> Requirements Table/1(ATR_GND_CTRL)
  ATR_PACE_CTRL/1 -> Requirements Table/2(ATR_PACE_CTRL)
  PACE_CHARGE_CTRL/1 -> Requirements Table/4(PACE_CHARGE_CTRL)
  PACE_GND_CTRL/1 -> Requirements Table/5(PACE_GND_CTRL)
  VENT_GND_CTRL/1 -> Requirements Table/6(VENT_GND_CTRL)
  VENT_PACE_CTRL/1 -> Requirements Table/7(VENT_PACE_CTRL)
  FRONTEND_CTRL/1 -> Requirements Table/3(FRONTEND_CTRL)
  PaceMakerMode/1 -> Requirements Table/8(mode)
  in_default/1 -> Requirements Table/9(in_default)

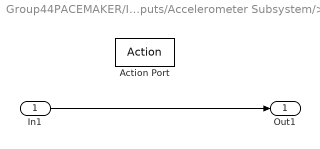
== system Group44PACEMAKER/Inputs/Accelerometer Subsystem/>7.9 ==
  In1 : Inport
  Action Port : ActionPort  ActionPortLabel=elseif(u1>7.9)
  Out1 : Outport
  wires:
  In1/1 -> Out1/1

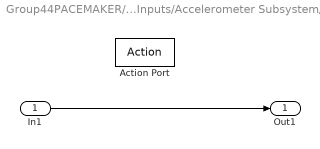
== system Group44PACEMAKER/Inputs/Accelerometer Subsystem/>8 ==
  In1 : Inport
  Action Port : ActionPort  ActionPortLabel=if(u1 > 8)
  Out1 : Outport
  wires:
  In1/1 -> Out1/1

== system Group44PACEMAKER/Inputs/Accelerometer Subsystem/Accelerometer ==
  FXOS8700 6-Axes Sensor : frdmk64flib/FXOS8700 6-Axes Sensor  Activesensor=Accelerometer only  ODR=800Hz  HybridODR=400Hz  Accelfullrange=-8g to +8g  SampleTime=-1
  Acceleration : Outport
  wires:
  FXOS8700 6-Axes Sensor/1 -> Acceleration/1

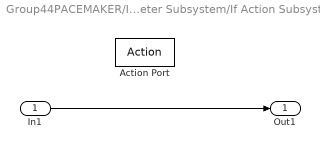
== system Group44PACEMAKER/Inputs/Accelerometer Subsystem/If Action Subsystem ==
  In1 : Inport
  Action Port : ActionPort  ActionPortLabel=elseif( u1>7.6)
  Out1 : Outport
  wires:
  In1/1 -> Out1/1

== system Group44PACEMAKER/Inputs/Accelerometer Subsystem/If Action Subsystem1 ==
  In1 : Inport
  Action Port : ActionPort  ActionPortLabel=elseif( u1>7.5)
  Out1 : Outport
  wires:
  In1/1 -> Out1/1

== system Group44PACEMAKER/Inputs/Accelerometer Subsystem/If Action Subsystem10 ==
  In1 : Inport
  Action Port : ActionPort  ActionPortLabel=elseif( u1>6.6)
  Out1 : Outport
  wires:
  In1/1 -> Out1/1

== system Group44PACEMAKER/Inputs/Accelerometer Subsystem/If Action Subsystem11 ==
  In1 : Inport
  Action Port : ActionPort  ActionPortLabel=elseif( u1>6.5)
  Out1 : Outport
  wires:
  In1/1 -> Out1/1

== system Group44PACEMAKER/Inputs/Accelerometer Subsystem/If Action Subsystem12 ==
  In1 : Inport
  Action Port : ActionPort  ActionPortLabel=elseif( u1>6.4)
  Out1 : Outport
  wires:
  In1/1 -> Out1/1

== system Group44PACEMAKER/Inputs/Accelerometer Subsystem/If Action Subsystem13 ==
  In1 : Inport
  Action Port : ActionPort  ActionPortLabel=elseif( u1>6.3)
  Out1 : Outport
  wires:
  In1/1 -> Out1/1

== system Group44PACEMAKER/Inputs/Accelerometer Subsystem/If Action Subsystem14 ==
  In1 : Inport
  Action Port : ActionPort  ActionPortLabel=elseif( u1>6.2)
  Out1 : Outport
  wires:
  In1/1 -> Out1/1

== system Group44PACEMAKER/Inputs/Accelerometer Subsystem/If Action Subsystem15 ==
  In1 : Inport
  Action Port : ActionPort  ActionPortLabel=elseif( u1>6.1)
  Out1 : Outport
  wires:
  In1/1 -> Out1/1

== system Group44PACEMAKER/Inputs/Accelerometer Subsystem/If Action Subsystem16 ==
  In1 : Inport
  Action Port : ActionPort  ActionPortLabel=elseif( u1 >6)
  Out1 : Outport
  wires:
  In1/1 -> Out1/1

== system Group44PACEMAKER/Inputs/Accelerometer Subsystem/If Action Subsystem17 ==
  In1 : Inport
  Action Port : ActionPort  ActionPortLabel=elseif( u1>5.9)
  Out1 : Outport
  wires:
  In1/1 -> Out1/1

== system Group44PACEMAKER/Inputs/Accelerometer Subsystem/If Action Subsystem18 ==
  In1 : Inport
  Action Port : ActionPort  ActionPortLabel=elseif( u1>5.8)
  Out1 : Outport
  wires:
  In1/1 -> Out1/1

== system Group44PACEMAKER/Inputs/Accelerometer Subsystem/If Action Subsystem19 ==
  In1 : Inport
  Action Port : ActionPort  ActionPortLabel=elseif( u1>5.7)
  Out1 : Outport
  wires:
  In1/1 -> Out1/1

== system Group44PACEMAKER/Inputs/Accelerometer Subsystem/If Action Subsystem2 ==
  In1 : Inport
  Action Port : ActionPort  ActionPortLabel=elseif( u1>7.4)
  Out1 : Outport
  wires:
  In1/1 -> Out1/1

== system Group44PACEMAKER/Inputs/Accelerometer Subsystem/If Action Subsystem20 ==
  In1 : Inport
  Action Port : ActionPort  ActionPortLabel=elseif( u1>5.6)
  Out1 : Outport
  wires:
  In1/1 -> Out1/1

== system Group44PACEMAKER/Inputs/Accelerometer Subsystem/If Action Subsystem21 ==
  In1 : Inport
  Action Port : ActionPort  ActionPortLabel=elseif( u1>5.5)
  Out1 : Outport
  wires:
  In1/1 -> Out1/1

== system Group44PACEMAKER/Inputs/Accelerometer Subsystem/If Action Subsystem22 ==
  In1 : Inport
  Action Port : ActionPort  ActionPortLabel=elseif( u1>5.4)
  Out1 : Outport
  wires:
  In1/1 -> Out1/1

== system Group44PACEMAKER/Inputs/Accelerometer Subsystem/If Action Subsystem23 ==
  In1 : Inport
  Action Port : ActionPort  ActionPortLabel=elseif( u1>5.3)
  Out1 : Outport
  wires:
  In1/1 -> Out1/1

== system Group44PACEMAKER/Inputs/Accelerometer Subsystem/If Action Subsystem24 ==
  In1 : Inport
  Action Port : ActionPort  ActionPortLabel=elseif( u1>5.2)
  Out1 : Outport
  wires:
  In1/1 -> Out1/1

== system Group44PACEMAKER/Inputs/Accelerometer Subsystem/If Action Subsystem25 ==
  In1 : Inport
  Action Port : ActionPort  ActionPortLabel=elseif( u1>5.1)
  Out1 : Outport
  wires:
  In1/1 -> Out1/1

== system Group44PACEMAKER/Inputs/Accelerometer Subsystem/If Action Subsystem26 ==
  In1 : Inport
  Action Port : ActionPort  ActionPortLabel=else
  Out1 : Outport
  wires:
  In1/1 -> Out1/1

== system Group44PACEMAKER/Inputs/Accelerometer Subsystem/If Action Subsystem3 ==
  In1 : Inport
  Action Port : ActionPort  ActionPortLabel=elseif( u1>7.3)
  Out1 : Outport
  wires:
  In1/1 -> Out1/1

== system Group44PACEMAKER/Inputs/Accelerometer Subsystem/If Action Subsystem4 ==
  In1 : Inport
  Action Port : ActionPort  ActionPortLabel=elseif( u1>7.2)
  Out1 : Outport
  wires:
  In1/1 -> Out1/1

== system Group44PACEMAKER/Inputs/Accelerometer Subsystem/If Action Subsystem5 ==
  In1 : Inport
  Action Port : ActionPort  ActionPortLabel=elseif( u1>7.1)
  Out1 : Outport
  wires:
  In1/1 -> Out1/1

== system Group44PACEMAKER/Inputs/Accelerometer Subsystem/If Action Subsystem6 ==
  In1 : Inport
  Action Port : ActionPort  ActionPortLabel=elseif( u1 > 7)
  Out1 : Outport
  wires:
  In1/1 -> Out1/1

== system Group44PACEMAKER/Inputs/Accelerometer Subsystem/If Action Subsystem7 ==
  In1 : Inport
  Action Port : ActionPort  ActionPortLabel=elseif( u1>6.9)
  Out1 : Outport
  wires:
  In1/1 -> Out1/1

== system Group44PACEMAKER/Inputs/Accelerometer Subsystem/If Action Subsystem8 ==
  In1 : Inport
  Action Port : ActionPort  ActionPortLabel=elseif( u1>6.8)
  Out1 : Outport
  wires:
  In1/1 -> Out1/1

== system Group44PACEMAKER/Inputs/Accelerometer Subsystem/If Action Subsystem9 ==
  In1 : Inport
  Action Port : ActionPort  ActionPortLabel=elseif( u1>6.7)
  Out1 : Outport
  wires:
  In1/1 -> Out1/1

== system Group44PACEMAKER/Inputs/Accelerometer Subsystem/Moderate activity LRL if subsystem ==
  In1 : Inport
  Action Port : ActionPort  ActionPortLabel=elseif( u1>7.8)
  Out1 : Outport
  wires:
  In1/1 -> Out1/1

== system Group44PACEMAKER/Inputs/Accelerometer Subsystem/RF == 1 ==
  In1 : Inport
  Action Port : ActionPort  ActionPortLabel=case [ 1 ]:
  Out1 : Outport
  wires:
  In1/1 -> Out1/1

== system Group44PACEMAKER/Inputs/Accelerometer Subsystem/RF == 10 ==
  In1 : Inport
  Action Port : ActionPort  ActionPortLabel=case [ 10 ]:
  Out1 : Outport
  wires:
  In1/1 -> Out1/1

== system Group44PACEMAKER/Inputs/Accelerometer Subsystem/RF == 11 ==
  In1 : Inport
  Action Port : ActionPort  ActionPortLabel=case [ 11 ]:
  Out1 : Outport
  wires:
  In1/1 -> Out1/1

== system Group44PACEMAKER/Inputs/Accelerometer Subsystem/RF == 12 ==
  In1 : Inport
  Action Port : ActionPort  ActionPortLabel=case [ 12 ]:
  Out1 : Outport
  wires:
  In1/1 -> Out1/1

== system Group44PACEMAKER/Inputs/Accelerometer Subsystem/RF == 13 ==
  In1 : Inport
  Action Port : ActionPort  ActionPortLabel=case [ 13 ]:
  Out1 : Outport
  wires:
  In1/1 -> Out1/1

== system Group44PACEMAKER/Inputs/Accelerometer Subsystem/RF == 14 ==
  In1 : Inport
  Action Port : ActionPort  ActionPortLabel=case [ 14 ]:
  Out1 : Outport
  wires:
  In1/1 -> Out1/1

== system Group44PACEMAKER/Inputs/Accelerometer Subsystem/RF == 15 ==
  In1 : Inport
  Action Port : ActionPort  ActionPortLabel=case [ 15 ]:
  Out1 : Outport
  wires:
  In1/1 -> Out1/1

== system Group44PACEMAKER/Inputs/Accelerometer Subsystem/RF == 16 ==
  In1 : Inport
  Action Port : ActionPort  ActionPortLabel=case [ 16 ]:
  Out1 : Outport
  wires:
  In1/1 -> Out1/1

== system Group44PACEMAKER/Inputs/Accelerometer Subsystem/RF == 2 ==
  In1 : Inport
  Action Port : ActionPort  ActionPortLabel=case [ 2 ]:
  Out1 : Outport
  wires:
  In1/1 -> Out1/1

== system Group44PACEMAKER/Inputs/Accelerometer Subsystem/RF == 3 ==
  In1 : Inport
  Action Port : ActionPort  ActionPortLabel=case [ 3 ]:
  Out1 : Outport
  wires:
  In1/1 -> Out1/1

== system Group44PACEMAKER/Inputs/Accelerometer Subsystem/RF == 4 ==
  In1 : Inport
  Action Port : ActionPort  ActionPortLabel=case [ 4 ]:
  Out1 : Outport
  wires:
  In1/1 -> Out1/1

== system Group44PACEMAKER/Inputs/Accelerometer Subsystem/RF == 5 ==
  In1 : Inport
  Action Port : ActionPort  ActionPortLabel=case [ 5 ]:
  Out1 : Outport
  wires:
  In1/1 -> Out1/1

== system Group44PACEMAKER/Inputs/Accelerometer Subsystem/RF == 6 ==
  In1 : Inport
  Action Port : ActionPort  ActionPortLabel=case [ 6 ]:
  Out1 : Outport
  wires:
  In1/1 -> Out1/1

== system Group44PACEMAKER/Inputs/Accelerometer Subsystem/RF == 7 ==
  In1 : Inport
  Action Port : ActionPort  ActionPortLabel=case [ 7 ]:
  Out1 : Outport
  wires:
  In1/1 -> Out1/1

== system Group44PACEMAKER/Inputs/Accelerometer Subsystem/RF == 8 ==
  In1 : Inport
  Action Port : ActionPort  ActionPortLabel=case [ 8 ]:
  Out1 : Outport
  wires:
  In1/1 -> Out1/1

== system Group44PACEMAKER/Inputs/Accelerometer Subsystem/RF == 9 ==
  In1 : Inport
  Action Port : ActionPort  ActionPortLabel=case [ 9 ]:
  Out1 : Outport
  wires:
  In1/1 -> Out1/1

== system Group44PACEMAKER/Inputs/Accelerometer Subsystem/Vigorous activity LRL if subsystem ==
  In1 : Inport
  Action Port : ActionPort  ActionPortLabel=elseif( u1>7.7)
  Out1 : Outport
  wires:
  In1/1 -> Out1/1

== stateflow chart Group44PACEMAKER/OutputPins & Requirements/Requirements Table Subsystem/Requirements Table ==
  (default) -> (junction 1073742542)
  (junction 1073742542) -> (junction 1073742543) : {
      | % SF_REQ_REV_07
      | }
  (junction 1073742543) -> (junction 1073742545) : {
      | % HEADER_ASSIGNMENTS
      |
      | }
  (junction 1073742545) -> (junction 1073742547) : {
      | % START_A_4
      | }
  (junction 1073742547) -> (junction 1073742549) : {
      | }
  (junction 1073742549) -> (junction 1073742551) : {
      | reqtable_assumption((t>=0), 4);
      | }
  (junction 1073742551) -> (junction 1073742553) : {
      | }
  (junction 1073742553) -> (junction 1073742555) : {
      | % END_A_4
      | }
  (junction 1073742555) -> (junction 1073742557) : {
      | % START_R_28
      | }
  (junction 1073742557) -> (junction 1073742559) : {
      | }
  (junction 1073742559) -> (junction 1073742561)
  (junction 1073742561) -> (junction 1073742563) [order 1] : [(((in_default) == (1))) && (((PACE_CHARGE_CTRL ) == (0)))]
  (junction 1073742561) -> (junction 1073742569) [order 2]
  (junction 1073742563) -> (junction 1073742565) : {
      | reqtable_postcondition((((ATR_PACE_CTRL ) == (0))) && (((VENT_PACE_CTRL ) == (0))) && (((ATR_GND_CTRL ) == (0))) && (((VENT_GND_CTRL ) == (0))) && (((PACE_GND_CTRL) == (0))), 'R:1');
      |
      |
      | }
  (junction 1073742565) -> (junction 1073742567) : {
      | }
  (junction 1073742567) -> (junction 1073742569)
  (junction 1073742569) -> (junction 1073742571)
  (junction 1073742571) -> (junction 1073742573) : {
      | % END_R_28
      | }
  (junction 1073742573) -> (junction 1073742575) : {
      | % START_R_1
      | }
  (junction 1073742575) -> (junction 1073742577) : {
      | }
  (junction 1073742577) -> (junction 1073742579)
  (junction 1073742579) -> (junction 1073742581) [order 1] : [(((in_default) == (0))) && (((PACE_CHARGE_CTRL ) == (1))) && (mode == "AOO" || mode == "AAI")]
  (junction 1073742579) -> (junction 1073742587) [order 2]
  (junction 1073742581) -> (junction 1073742583) : {
      | reqtable_postcondition((((ATR_PACE_CTRL ) == (0))) && (((VENT_PACE_CTRL ) == (0))) && (((ATR_GND_CTRL ) == (1))) && (((VENT_GND_CTRL ) == (0))) && (((PACE_GND_CTRL) == (1))), 'R:2');
      |
      |
      | }
  (junction 1073742583) -> (junction 1073742585) : {
      | }
  (junction 1073742585) -> (junction 1073742587)
  (junction 1073742587) -> (junction 1073742589)
  (junction 1073742589) -> (junction 1073742591) : {
      | % END_R_1
      | }
  (junction 1073742591) -> (junction 1073742593) : {
      | % START_R_25
      | }
  (junction 1073742593) -> (junction 1073742595) : {
      | }
  (junction 1073742595) -> (junction 1073742597)
  (junction 1073742597) -> (junction 1073742599) [order 1] : [(((in_default) == (0))) && (((PACE_CHARGE_CTRL ) == (1))) && (mode == "VOO" || mode == "VVI")]
  (junction 1073742597) -> (junction 1073742605) [order 2]
  (junction 1073742599) -> (junction 1073742601) : {
      | reqtable_postcondition((((ATR_PACE_CTRL ) == (0))) && (((VENT_PACE_CTRL ) == (0))) && (((ATR_GND_CTRL ) == (0))) && (((VENT_GND_CTRL ) == (1))) && (((PACE_GND_CTRL) == (1))), 'R:3');
      |
      |
      | }
  (junction 1073742601) -> (junction 1073742603) : {
      | }
  (junction 1073742603) -> (junction 1073742605)
  (junction 1073742605) -> (junction 1073742607)
  (junction 1073742607) -> (junction 1073742609) : {
      | % END_R_25
      | }
  (junction 1073742609) -> (junction 1073742611) : {
      | % START_R_10
      | }
  (junction 1073742611) -> (junction 1073742613) : {
      | }
  (junction 1073742613) -> (junction 1073742615)
  (junction 1073742615) -> (junction 1073742617) [order 1] : [(((in_default) == (0))) && (((PACE_CHARGE_CTRL ) == (0))) && (mode == "AOO" || mode == "AAI")]
  (junction 1073742615) -> (junction 1073742623) [order 2]
  (junction 1073742617) -> (junction 1073742619) : {
      | reqtable_postcondition((((ATR_PACE_CTRL ) == (1))) && (((VENT_PACE_CTRL ) == (0))) && (((ATR_GND_CTRL ) == (0))) && (((VENT_GND_CTRL ) == (0))) && (((PACE_GND_CTRL) == (1))), 'R:4');
      |
      |
      | }
  (junction 1073742619) -> (junction 1073742621) : {
      | }
  (junction 1073742621) -> (junction 1073742623)
  (junction 1073742623) -> (junction 1073742625)
  (junction 1073742625) -> (junction 1073742627) : {
      | % END_R_10
      | }
  (junction 1073742627) -> (junction 1073742629) : {
      | % START_R_19
      | }
  (junction 1073742629) -> (junction 1073742631) : {
      | }
  (junction 1073742631) -> (junction 1073742633)
  (junction 1073742633) -> (junction 1073742635) [order 1] : [(((in_default) == (0))) && (((PACE_CHARGE_CTRL ) == (0))) && (mode == "VOO" || mode == "VVI")]
  (junction 1073742633) -> (junction 1073742641) [order 2]
  (junction 1073742635) -> (junction 1073742637) : {
      | reqtable_postcondition((((ATR_PACE_CTRL ) == (0))) && (((VENT_PACE_CTRL ) == (1))) && (((ATR_GND_CTRL ) == (0))) && (((VENT_GND_CTRL ) == (0))) && (((PACE_GND_CTRL) == (1))), 'R:5');
      |
      |
      | }
  (junction 1073742637) -> (junction 1073742639) : {
      | }
  (junction 1073742639) -> (junction 1073742641)
  (junction 1073742641) -> (junction 1073742643)
  (junction 1073742643) -> (junction 1073742645) : {
      | % END_R_19
      | }
  (junction 1073742645) -> (junction 1073742647) : {
      | % START_R_13
      | }
  (junction 1073742647) -> (junction 1073742649) : {
      | }
  (junction 1073742649) -> (junction 1073742651)
  (junction 1073742651) -> (junction 1073742653) [order 1] : [(((in_default) == (0))) && (((FRONTEND_CTRL ) == (1))) && (mode == "AAI" || mode == "VVI")]
  (junction 1073742651) -> (junction 1073742659) [order 2]
  (junction 1073742653) -> (junction 1073742655) : {
      | reqtable_postcondition((((ATR_PACE_CTRL ) == (0))) && (((VENT_PACE_CTRL ) == (0))) && (((PACE_GND_CTRL) == (1))), 'R:6');
      |
      |
      | }
  (junction 1073742655) -> (junction 1073742657) : {
      | }
  (junction 1073742657) -> (junction 1073742659)
  (junction 1073742659) -> (junction 1073742661)
  (junction 1073742661) -> (junction 1073742663) : {
      | % END_R_13
      | }
  data: ATR_GND_CTRL input boolean; ATR_PACE_CTRL input boolean; FRONTEND_CTRL input boolean; PACE_CHARGE_CTRL input boolean; PACE_GND_CTRL input boolean; VENT_GND_CTRL input boolean; VENT_PACE_CTRL input boolean; mode input string; in_default input boolean

== stateflow chart Group44PACEMAKER/Inputs/Accelerometer Subsystem/Change LRL Smoothly ==
  state Raise_HeartRate
    entry:
    outputLRL = currLRL
  state Increment_currLRL_Down
    entry:
    currLRL = currLRL - rate_of_change
  state Speed_Up_HeartRate
    entry:
    rate_of_change = (outputLRL-inputLRL)/(reaction_time*10) *(2-(Response_factor/100))
    %Says how many seconds I need to decrease the LRL per tenth of a second passed in the simulation
    currLRL = outputLRL %setting the step change LRL to its starting point
    setPoint = inputLRL
  state Wait_For_Change
    entry:
    outputLRL = inputLRL;
  state Slow_Down_HeartRate
    entry:
    rate_of_change = (inputLRL - outputLRL)/(recovery_time*60*10) *(2-(Response_factor/100))
    %how many seconds to increase the LRL by for each tenth of a second passed in the simulation
    %reaction time is in minutes
    currLRL = outputLRL
    setPoint = inputLRL
  state Increment_currLRL_Up
    entry:
    currLRL = currLRL + rate_of_change
  state Start_Here
    entry:
    outputLRL = 1000 %no LRL has been set to the heart yet so we'll start off at 60 bpm
  state Lower_HeartRate
    entry:
    outputLRL = currLRL
  Raise_HeartRate -> (junction 54) [order 2] : [outputLRL > inputLRL]
  Raise_HeartRate -> (junction 51) [order 1] : [outputLRL <= inputLRL]
  (junction 54) -> Increment_currLRL_Down [order 2] : [setPoint == inputLRL]
  (junction 54) -> Speed_Up_HeartRate [order 1] : [setPoint ~= inputLRL]
  Increment_currLRL_Down -> Raise_HeartRate : after(100,msec)
  Speed_Up_HeartRate -> Increment_currLRL_Down
  (junction 51) -> Speed_Up_HeartRate [order 1] : [outputLRL>inputLRL]
  (junction 51) -> Wait_For_Change [order 2] : [outputLRL <= inputLRL+0.1 && outputLRL >= inputLRL-0.1]
  Wait_For_Change -> (junction 51)
  (junction 51) -> Slow_Down_HeartRate [order 3] : [outputLRL<inputLRL]
  Lower_HeartRate -> (junction 51) [order 1] : [outputLRL >= inputLRL]
  Start_Here -> (junction 51)
  (junction 64) -> Slow_Down_HeartRate [order 2] : [setPoint ~= inputLRL]
  Slow_Down_HeartRate -> Increment_currLRL_Up
  (junction 64) -> Increment_currLRL_Up [order 1] : [setPoint == inputLRL]
  Increment_currLRL_Up -> Lower_HeartRate : after(100,msec)
  Lower_HeartRate -> (junction 64) [order 2] : [outputLRL < inputLRL]
  (default) -> Start_Here
  data: Response_factor input; inputLRL input; reaction_time input; recovery_time input; currLRL local; outputLRL output; rate_of_change local; setPoint local
